simulink model "send_pwm"  (R2023a)
settings: Solver=FixedStepAuto  StartTime=0.0  StopTime=Inf  FixedStep=0.01  RelTol=1e-3
libraries: realtime_pacer_lib x2, dspnetwork x1
settings Model: PacingRate=10  Creator=main  LastModifiedBy=Dell

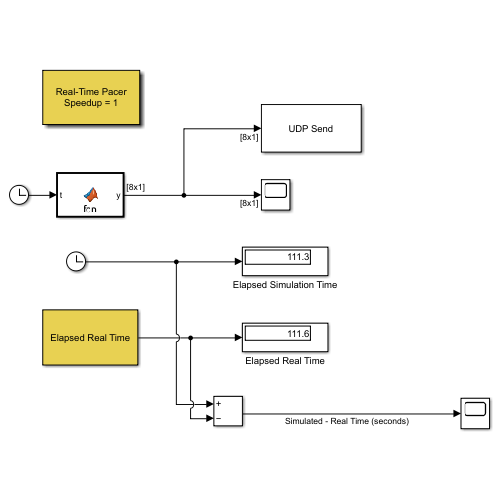
[thumbnail: Simulink's stored preview of the top-level diagram]
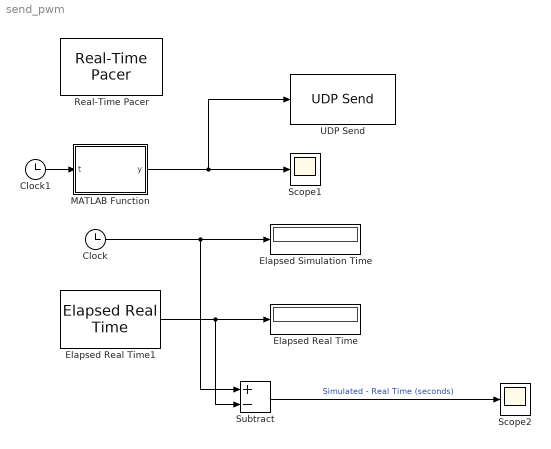
== system send_pwm ==
  Clock : Clock
  Clock1 : Clock
  Elapsed Real Time : Display
      settings: Decimation=2
  Elapsed Real Time1 : realtime_pacer_lib/Elapsed Real Time
  Elapsed Simulation Time : Display
      settings: Decimation=2
  MATLAB Function : MATLAB Function  TreatAsAtomicUnit=on
  Real-Time Pacer : realtime_pacer_lib/Real-Time Pacer  simTimePerRealTime=1
  Scope1 : Scope
  Scope2 : Scope
  Subtract : Sum  Inputs=+-
  UDP Send : dspnetwork/UDP Send  remoteURL='192.168.1.153'  remotePort=5000  localURL='0.0.0.0'  localPortSource=Automatically determine  localPort=-1  sendBufferSize=64  sampletime=-1  blockPlatform=[]  separateLengthPort=0
      settings: LibrarySourceBlock=dspsnks4/UDP Send
  wires:
  Clock/1 -> Elapsed Simulation Time/1, Subtract/1
  MATLAB Function/1(y) -> UDP Send/1, Scope1/1
  Elapsed Real Time1/1 -> Elapsed Real Time/1, Subtract/2
  Subtract/1 -> Scope2/1  "Simulated - Real Time (seconds)"
  Clock1/1 -> MATLAB Function/1(t)

== matlab function send_pwm/MATLAB Function ==
  data: t input; y output
function y = fcn(t)

A = (0.5:0.5:4)';
% phase = [   0.915735525189067; 0.792207329559554; 0.959492426392903; 0.655740699156587; 0.035711678574190; 0.849129305868777; 0.933993247757551; 0.678735154857773];
phase = zeros(8,1);
y = A.*sin(ones(8,1)*t-phase);
